simulink model "Simulink_Simulation"  (R2022b)
settings: Solver=FixedStepAuto  StartTime=0.0  StopTime=30  FixedStep=5e-4  RelTol=1e-3
values from neighbouring files (symbols this model uses):
  Kd_PitchRate_val = 2    [Simscape_Simulation_Init.m]
  Kd_RollRate_val = 3    [Simscape_Simulation_Init.m]
  Kd_YawRate_val = 0e6    (= 0)    [Simscape_Simulation_Init.m]
  Ki_PitchRate_val = 7    [Simscape_Simulation_Init.m]
  Ki_RollRate_val = 7    [Simscape_Simulation_Init.m]
  Ki_Thrust_val = 200e6    (= 200000000)    [Simscape_Simulation_Init.m]
  Ki_YawRate_val = 100e6    (= 100000000)    [Simscape_Simulation_Init.m]
  Kp_PitchRate_val = 20    [Simscape_Simulation_Init.m]
  Kp_RollRate_val = 25    [Simscape_Simulation_Init.m]
  Kp_Thrust_val = 2e6    (= 2000000)    [Simscape_Simulation_Init.m]
  Kp_YawRate_val = 110e6    (= 110000000)    [Simscape_Simulation_Init.m]
  Kq_PitchRate_val = 4    [Simscape_Simulation_Init.m]
  Kr_YawRate_val = 7    [Simscape_Simulation_Init.m]
  N_PitchRate_val = 20    [Simscape_Simulation_Init.m]
  N_YawRate_val = 20    [Simscape_Simulation_Init.m]
  Ts_val = 0.01    [Simscape_Simulation_Init.m]
undefined symbols (not defined in the file or in its folder): DiscIntNeverNeededParam, smiData, X, Y, Z
libraries: sm_lib x27, nesl_utility x14, slpidlib x2, simulink x1
(part 2 of 2)

== system Simulink_Simulation/Aircraft Dynamics/Subsystem/X1_THORN_BODY_SIMSCAPE_1_RIGID ==
  ReferenceFrame : sm_lib/Frames and Transforms/Reference Frame
  Solid : sm_lib/Body Elements/File Solid  ExtGeomFileName=X1_THORN_BODY_SIMSCAPE_Predeterminado_sldprt.STEP  UnitType=FromFile  ExtGeomFileUnits=m  StepReaderType=HEX  ExportConvexHullGeometry=off  InertiaType=Custom  Mass=1172  MassUnits=g  CenterOfMass=[0, 0, 0]  CenterOfMassUnits=mm  MomentsOfInertia=[3100.52, 5691.13, 8307.11]  MomentsOfInertiaUnits=kg*mm^2  ProductsOfInertia=[0,0,0]  ProductsOfInertiaUnits=kg*mm^2  BasedOnType=DensityFromFile  Density=1000  DensityUnits=kg/m^3  DoExposeReferenceFrame=on  SerializedFrames=<Frames/>  GraphicType=FromGeometry  MarkerShape=Sphere  MarkerSize=10  GraphicVisPropType=SimpleVisualProperties  GraphicDiffuseColor=smiData.Solid(1).color  GraphicSpecularColor=[0.5 0.5 0.5 1.0]  GraphicAmbientColor=[0.15 0.15 0.15 1.0]  GraphicEmissiveColor=[0.0 0.0 0.0 1.0]  GraphicShininess=75  GraphicOpacity=smiData.Solid(1).opacity
  Transform : sm_lib/Frames and Transforms/Rigid Transform  TranslationMethod=Cartesian  TranslationStandardOffset=0  TranslationLengthUnit=mm  TranslationStandardAxis=+Z  TranslationCartesianOffset=smiData.RigidTransform(1).translation  TranslationROffset=0  TranslationROffsetUnits=m  TranslationZOffset=0  TranslationZOffsetUnits=m  TranslationThetaOffset=0  TranslationThetaOffsetUnits=deg  RotationMethod=ArbitraryAxis  RotationAngleUnits=rad  RotationStandardAxis=+Z  RotationAngle=smiData.RigidTransform(1).angle  RotationArbitraryAxis=smiData.RigidTransform(1).axis  FollAlignAxisA=+X  BaseAlignAxisA=+Y  FollAlignAxisB=+Y  BaseAlignAxisB=+Z  RotationSequenceAxes=FollowerAxes  RotationSequence=XYX  RotationSequenceAngles=[0 0 0]  RotationSequenceAnglesUnits=deg  RotationMatrix=[1 0 0; 0 1 0; 0 0 1]  Quaternion=[1 0 0 0]
  Transform1 : sm_lib/Frames and Transforms/Rigid Transform  TranslationMethod=Cartesian  TranslationStandardOffset=0  TranslationLengthUnit=mm  TranslationStandardAxis=+Z  TranslationCartesianOffset=smiData.RigidTransform(3).translation  TranslationROffset=0  TranslationROffsetUnits=m  TranslationZOffset=0  TranslationZOffsetUnits=m  TranslationThetaOffset=0  TranslationThetaOffsetUnits=deg  RotationMethod=ArbitraryAxis  RotationAngleUnits=rad  RotationStandardAxis=+Z  RotationAngle=smiData.RigidTransform(3).angle  RotationArbitraryAxis=smiData.RigidTransform(3).axis  FollAlignAxisA=+X  BaseAlignAxisA=+Y  FollAlignAxisB=+Y  BaseAlignAxisB=+Z  RotationSequenceAxes=FollowerAxes  RotationSequence=XYX  RotationSequenceAngles=[0 0 0]  RotationSequenceAnglesUnits=deg  RotationMatrix=[1 0 0; 0 1 0; 0 0 1]  Quaternion=[1 0 0 0]
  F2 : PMIOPort  Side=Left
  F1 : PMIOPort  Port=2  Side=Right
  F : PMIOPort  Port=3  Side=Right
  connections:
  Solid/RConn1 -- ReferenceFrame/RConn1 -- Transform/LConn1 -- Transform1/LConn1 -- F2/RConn1
  Transform/RConn1 -- F/RConn1
  Transform1/RConn1 -- F1/RConn1

== matlab function Simulink_Simulation/Aircraft Dynamics/Thrust Vectoring Forces/MATLAB Function ==
  data: omega1 input; Tx_ctrl output; omega2 input; alfa1 input; alfa2 input; Ty_ctrl output; Tz_ctrl output; Mx_ctrl output; My_ctrl output; Mz_ctrl output
function [Tx_ctrl, Ty_ctrl, Tz_ctrl, Mx_ctrl, My_ctrl, Mz_ctrl] = fcn(omega1, omega2, alfa1, alfa2)

%% Compute Forces based on inputs

% Test Stand Constants

setpoint_R = 1480; % Servo setpoint (neutral 0 deg)
setpoint_L = 1400;

A_Tx = 3.45e-8 / 2.7; % Compensar que esta en el dron
B_Tx = 3e-3 * 0.1 / 0.09; % Compensar el nou servo

A_Tz = -1.0e-8 / 2.7; % Compensar que esta en el dron
B_Tz = 7e-3 * 0.1 / 0.09; % Compensar el nou servo

A_My = -1.3e-9 / 2.7; % Compensar que esta en el dron (invent total tenint en compte una mica que el dron s'enlairava a partir de les 22000 rpms)
B_My = 8e-3 * 0.1 / 0.09; % Compensar el nou servo

% Thrust calculation

Tx_R = A_Tx*omega1^2*cos((alfa1-setpoint_R)*B_Tx);
Tz_R = A_Tz*omega1^2*sin((alfa1-setpoint_R)*B_Tz);
My_R = A_My*omega1^2*sin((alfa1-setpoint_R)*B_My);

Tx_L = A_Tx*omega2^2*cos((alfa2-setpoint_L)*B_Tx);
Tz_L = A_Tz*omega2^2*sin((alfa2-setpoint_L)*B_Tz);
My_L = A_My*omega2^2*sin((alfa2-setpoint_L)*B_My);

% Airframe parameters

x_CoG = 33.82e-3; % m
z_CoG = 0.34e-3; % m
lt_x = 60e-3; % m
lt_y = 80e-3; % m

% Control forces calculation

Tx_ctrl = Tx_R + Tx_L;
Ty_ctrl = 0;
Tz_ctrl = Tz_R - Tz_L;

Mx_ctrl = (Tz_R + Tz_L) * lt_y;
My_ctrl = My_R - My_L - (Tx_L + Tx_R) * z_CoG + (Tz_R * (x_CoG - lt_x)) - (Tz_L * (x_CoG - lt_x));
Mz_ctrl = (Tx_L - Tx_R) * lt_y;

== matlab function Simulink_Simulation/Attitude Controller/Reference Generator ==
  data: q0 input; p_error output; q1 input; q2 input; q3 input; pitch input; yaw input; q_error output; r_error output
function [p_error,q_error,r_error] = fcn(q0, q1, q2, q3, pitch, yaw)

vec_x_World = [0;0;1];

q_curr = [q0;q1;q2;q3];

vec_y_Aircraft = [2*(q1*q2 - q0*q3); 1 - 2*(q1^2 + q3^2); 2*(q2*q3 + q0*q1)];


vec_z_World = cross(vec_x_World,vec_y_Aircraft);
vec_y_World = cross(vec_z_World,vec_x_World);


%% 3) Build base rotation matrix R0 = [x_w, y_w, z_w]
R0 = [vec_x_World, vec_y_World, vec_z_World];

%% 4) Build small rotations about world-frame X then Y
  
Ry = [ cos(pitch), 0, sin(pitch);
             0, 1,       0;
      -sin(pitch), 0, cos(pitch)];


Rz = [cos(yaw), -sin(yaw), 0 ;
      sin(yaw), cos(yaw),  0 ;
      0,      0,           1];

% Composite: first yaw (Ry), then roll (Ry) in the *body frame*
R_ref = R0 * Ry * Rz;

%% 5) Convert R_ref into quaternion [q0_ref q1_ref q2_ref q3_ref]
q_ref = rotm2quat(R_ref)';  % returns [w x y z]

if dot([q0,q1,q2,q3], q_ref) < 0

    q_ref = -q_ref;
end

% q0, q1 are 4×1 [q0; qv] quaternions (scalar-first)
dq = (q_ref - q_curr);

% build the 4×3 matrix M = [Ω(e1)q0, Ω(e2)q0, Ω(e3)q0]
e = eye(3);
M = zeros(4,3);
for i = 1:3
    M(:,i) = Omega(e(i,:)) * q_curr;
end

omega = 2*(M \ dq);   % least-squares if slightly overdetermined
p_error = omega(1);
q_error = omega(2);
r_error = omega(3);






function O = Omega(w)
    % returns the 4×4 Ω(w) matrix for quaternion kinematics
    p = w(1); q = w(2); r = w(3);
    O = [  0, -p, -q, -r;
           p,  0,  r, -q;
           q, -r,  0,  p;
           r,  q, -p,  0 ];
end

end

== matlab function Simulink_Simulation/Attitude Controller/MATLAB Function ==
  data: Aileron input; servo_R output; Elevator input; Rudder input; omega_squared input; servo_L output; omega_R output; omega_L output
function [servo_R, servo_L, omega_R, omega_L] = fcn(Aileron, Elevator, Rudder, omega_squared)

if (omega_squared/2 - Rudder) < 0

    omega_R = 0;
else

    omega_R = sqrt(omega_squared/2 - Rudder);
end


if (omega_squared/2 + Rudder) < 0

    omega_L = 0;
else
    
    omega_L = sqrt(omega_squared/2 + Rudder);
end

servo_R = -Aileron - Elevator;
servo_L = -Aileron + Elevator;
